simulink model "ball_and_beam_response"  (R2016a)
settings: Solver=VariableStepAuto  StartTime=0.0  StopTime=10.0  MaxStep=1e-3  RelTol=1e-3
settings Model: Creator=mgreiff  LastModifiedBy=mgreiff

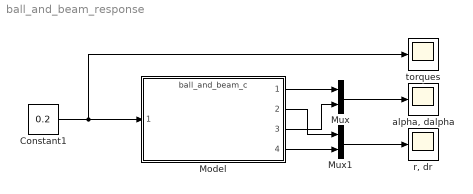
== system ball_and_beam_response ==
  Constant1 : Constant  Value=0.2
  Model : ModelReference  ModelNameDialog=ball_and_beam_c.slx  SimulationMode=Normal  ModelReferenceVersion=1.38
  Mux : Mux  Inputs=2
  Mux1 : Mux  Inputs=2
  "alpha, dalpha" : Scope
  "r, dr" : Scope
  torques : Scope
  wires:
  Model/1 -> Mux/1
  Model/3 -> Mux/2
  Model/4 -> Mux1/2
  Constant1/1 -> torques/1, Model/1
  Model/2 -> Mux1/1
  Mux1/1 -> "r, dr"/1
  Mux/1 -> "alpha, dalpha"/1
